simulink model "Prac3_setup"  (R2020a)
settings: Solver=VariableStepAuto  StartTime=0.0  StopTime=10.0  RelTol=1e-3
values from neighbouring files (symbols this model uses):
  prac3_param1 = 10.0595705167    [Prac3_paramaters007.mat]
  prac3_param2 = 0.01    [Prac3_paramaters007.mat]
  prac3_param3 = 0.17097230168    [Prac3_paramaters007.mat]
  prac3_param4 = 100    [Prac3_paramaters007.mat]
  prac3_param5 = 0.845451626268    [Prac3_paramaters007.mat]
  prac3_param6 = 0.01    [Prac3_paramaters007.mat]
settings Model: Creator=mluser  LastModifiedBy=mluser

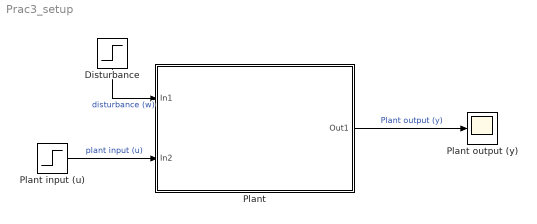
== system Prac3_setup ==
  Disturbance : Step  Time=5  After=0  SampleTime=0
  Plant : Subsystem
  Plant input (u) : Step  SampleTime=0
  Plant output (y) : Scope
  wires:
  Disturbance/1 -> Plant/1(In1)  "disturbance (w)"
  Plant input (u)/1 -> Plant/2(In2)  "plant input (u)"
  Plant/1(Out1) -> Plant output (y)/1  "Plant output (y)"

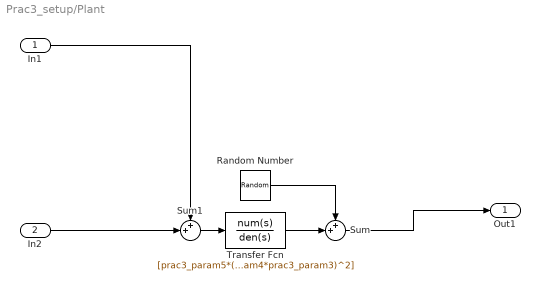
== system Prac3_setup/Plant ==
  In1 : Inport
  In2 : Inport  Port=2
  Random Number : RandomNumber  Variance=prac3_param6^2  SampleTime=0.001
  Sum : Sum  Inputs=++|
  Sum1 : Sum  Inputs=++|
  Transfer Fcn : TransferFcn  Numerator=[prac3_param5*(prac3_param4*prac3_param3)^2]  Denominator=[1 2*prac3_param4*prac3_param3*prac3_param2*prac3_param1 (prac3_param4*prac3_param3)^2]
  Out1 : Outport
  wires:
  Sum/1 -> Out1/1
  Transfer Fcn/1 -> Sum/2
  In2/1 -> Sum1/2
  In1/1 -> Sum1/1
  Sum1/1 -> Transfer Fcn/1
  Random Number/1 -> Sum/1
